simulink model "ACCmpr_DD"  (R2016b)
settings: configuration reference "CodeGenConfigSet" (kept outside this file)
values from neighbouring files (symbols this model uses):
  AirC_stCmprPsDiaDisbl_C = Calibration.Parameter    [init_ACCmpr_DD.m]
  AirC_stCmprPsDisbl_C = Calibration.Parameter    [init_ACCmpr_DD.m]
  SigTst_stACCmpr_C = Calibration.Parameter    [init_ACCmpr_DD.m]
  SigTst_swtACCmpr_C = Calibration.Parameter    [init_ACCmpr_DD.m]
undefined symbols (not defined in the file or in its folder): Switch_conv
libraries: simulink x4
settings Model: Creator=胡炎林  LastModifiedBy=liutao
settings ConfigSetRef: SourceLocation=Base Workspace

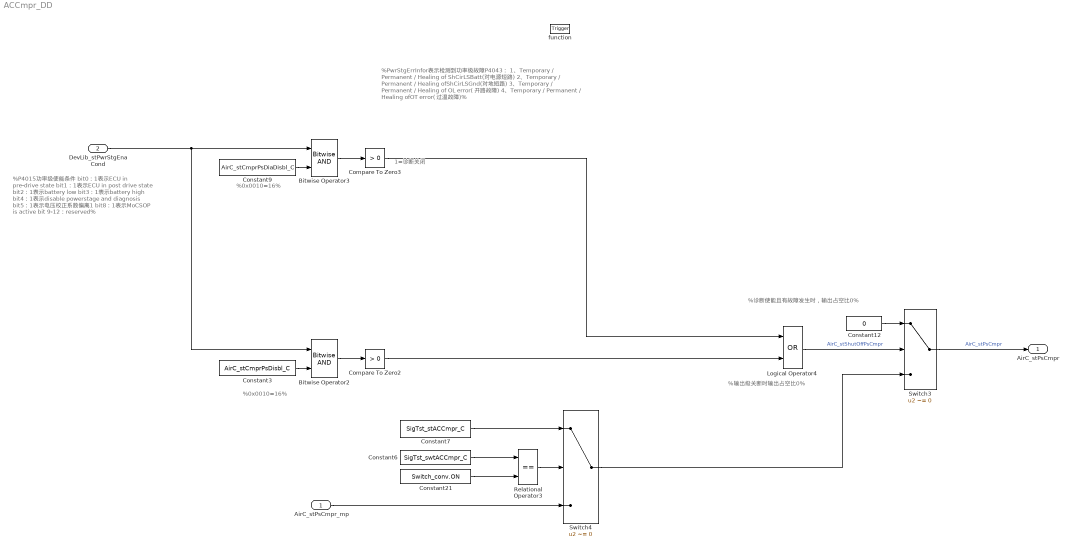
== system ACCmpr_DD ==
  note: 1=诊断关闭
  note: %0x0010=16%
  note: %PwrStgErrInfor表示检测到功率级故障P4043：
      | 1、Temporary / Permanent / Healing of ShCirLSBatt(对电源短路)
      | 2、Temporary / Permanent / Healing ofShCirLSGnd(对地短路)
      | 3、Temporary / Permanent / Healing of OL error(开路故障)
      | 4、Temporary / Permanent / Healing ofOT error(过温故障)%
  note: %P4015功率级使能条件
      | bit0：1表示ECU in pre-drive state
      | bit1：1表示ECU in post drive state
      | bit2：1表示battery low
      | bit3：1表示battery high
      | bit4：1表示disable powerstage and diagnosis
      | bit5：1表示电压校正系数偏离1
      | bit8：1表示MoCSOP is active
      | bit 9-12：reserved%
  note: %0x0010=16%
  note: %输出级关断时输出占空比0%
  note: %诊断使能且有故障发生时，输出占空比0%
  AirC_stPsCmpr_mp : Inport  Description=Measuring point for the digital output to the ACompressor actuator before error handling  OutMin=0  OutMax=1  OutDataTypeStr=boolean
  DevLib_stPwrStgEnaCond : Inport  Description=Control unit status relevant to power stage deactivation/error diagnosis  Port=2  OutMin=0  OutMax=65535  OutDataTypeStr=State_uint16
  function : TriggerPort  TriggerType=function-call  VariantControl=Variant
  Bitwise Operator2 : simulink/Logic and Bit Operations/Bitwise Operator  logicop=AND  UseBitMask=off  NumInputPorts=2  BitMask=bin2dec('00001111')  BitMaskRealWorld=Stored Integer
  Bitwise Operator3 : simulink/Logic and Bit Operations/Bitwise Operator  logicop=AND  UseBitMask=off  NumInputPorts=2  BitMask=bin2dec('00010000')  BitMaskRealWorld=Stored Integer
  Compare To Zero2 : simulink/Logic and Bit Operations/Compare To Zero  relop=>  OutDataTypeStr=boolean
  Compare To Zero3 : simulink/Logic and Bit Operations/Compare To Zero  relop=>  OutDataTypeStr=uint8
  Constant12 : Constant  Value=0  OutDataTypeStr=Inherit: Inherit via back propagation
  Constant21 : Constant  Value=Switch_conv.ON
  Constant3 : Constant  Value=AirC_stCmprPsDisbl_C
  Constant6 : Constant  Value=SigTst_swtACCmpr_C
  Constant7 : Constant  Value=SigTst_stACCmpr_C
  Constant9 : Constant  Value=AirC_stCmprPsDiaDisbl_C
  Logical Operator4 : Logic  Operator=OR  AllPortsSameDT=off  OutDataTypeStr=boolean
  Relational Operator3 : RelationalOperator  Operator===  OutDataTypeStr=boolean  RndMeth=Nearest
  Switch3 : Switch  Criteria=u2 ~= 0  OutDataTypeStr=Inherit: Inherit via back propagation  SaturateOnIntegerOverflow=on  InputSameDT=on
  Switch4 : Switch  Criteria=u2 ~= 0  SaturateOnIntegerOverflow=on  InputSameDT=on
  AirC_stPsCmpr : Outport  Description=Final digital output to the power stage of AC compressor actuator  OutMin=0  OutMax=1  OutDataTypeStr=boolean
  wires:
  Bitwise Operator3/1 -> Compare To Zero3/1
  Constant6/1 -> Relational Operator3/1
  Relational Operator3/1 -> Switch4/2
  Constant7/1 -> Switch4/1
  AirC_stPsCmpr_mp/1 -> Switch4/3
  Logical Operator4/1 -> Switch3/2  "AirC_stShutOffPsCmpr"
  Switch3/1 -> AirC_stPsCmpr/1  "AirC_stPsCmpr"
  Switch4/1 -> Switch3/3
  Constant9/1 -> Bitwise Operator3/2
  Constant3/1 -> Bitwise Operator2/2
  Compare To Zero2/1 -> Logical Operator4/2
  Constant21/1 -> Relational Operator3/2
  Constant12/1 -> Switch3/1
  Bitwise Operator2/1 -> Compare To Zero2/1
  DevLib_stPwrStgEnaCond/1 -> Bitwise Operator3/1, Bitwise Operator2/1
  Compare To Zero3/1 -> Logical Operator4/1
